simulink model "controllerTest"  (R2022b)
settings: Solver=ode45  StartTime=0  StopTime=T_f  MaxStep=MaxStep  RelTol=RelTol  AbsTol=1e-6
values from neighbouring files (symbols this model uses):
  A_ctrl = R_lti.A    [p62_inverted_pendulum.m]
  B_ctrl = R_lti.B    [p62_inverted_pendulum.m]
  beta = 0.1    [p62_inverted_pendulum.m]
  C_ctrl = R_lti.C    [p62_inverted_pendulum.m]
  D_ctrl = R_lti.D    [p62_inverted_pendulum.m]
  g = 9.81    [p62_inverted_pendulum.m]
  J_G = 0.006    [p62_inverted_pendulum.m]
  k = 0    [p62_inverted_pendulum.m]
  l = 0.6    [p62_inverted_pendulum.m]
  m = 0.2    [p62_inverted_pendulum.m]
  M = 0.5    [p62_inverted_pendulum.m]
  omega0 = 0    [p62_inverted_pendulum.m]
  theta0 = deg2rad(45)    [p62_inverted_pendulum.m]
  theta_ref = 0    [p62_inverted_pendulum.m]
  v0 = 0    [p62_inverted_pendulum.m]
  x0 = -5    [p62_inverted_pendulum.m]
Description:
  | Inverted Pendulum with Animation
  | 
  | This example shows how to model an inverted pendulum.  The animation is created using MATLAB(R) Handle Graphics(R).  The animation block is a masked
  | S-function.  For more information, use the context menu to look under the Animation block's mask
  | and open the S-function for editing.
settings Model: Creator=The MathWorks, Inc.  LastModifiedBy=alessandro
settings SolverCC: AutoScaleAbsTol=off  AlgebraicLoopSolver=TrustRegion
settings DataIOCC: ExternalInput=[]  InitialState=[]  SaveFormat=Array  SaveOutput=off  SaveTime=off  ReturnWorkspaceOutputs=off
settings OptimizationCC: BlockReduction=off  BooleanDataType=off  ExpressionDepthLimit=2147483647  InitFltsAndDblsToZero=on  LifeSpan=inf
settings DebuggingCC: SaveWithParameterizedLinksMsg=none  UnderspecifiedInitializationDetection=Classic  MergeDetectMultiDrivingBlocksExec=none  SignalResolutionControl=TryResolveAllWithWarning  MultiTaskDSMMsg=warning  MultiTaskCondExecSysMsg=none  SigSpecEnsureSampleTimeMsg=none  FcnCallInpInsideContextMsg=warning  UnconnectedInputMsg=warning  UnconnectedOutputMsg=warning  UnconnectedLineMsg=warning  StateNameClashWarn=warning  SFUnexpectedBacktrackingDiag=warning  SFNoUnconditionalDefaultTransitionDiag=warning  SFExecutionAtInitializationDiag=none  SFMachineParentedDataDiag=warning  ArithmeticOperatorsInVariantConditions=warning
settings HardwareCC: ProdBitPerPointer=32  ProdBitPerSizeT=32  ProdBitPerPtrDiffT=32  ProdLargestAtomicFloat=None  ProdIntDivRoundTo=Undefined  ProdEndianess=Unspecified  ProdWordSize=32  ProdHWDeviceType=32-bit Generic  TargetUnknown=on
settings ModelReferenceCC: EnableRefExpFcnMdlSchedulingChecks=on  PropagateSignalLabelsOutOfModel=off
settings SFSimCC: SimUseLocalCustomCode=off  CustomCodeUndefinedFunction=UseInterfaceOnly
settings RTWCC: RTWUseLocalCustomCode=off
settings CodeAppCC: StateflowObjectComments=on
settings GRTTargetCC: TargetFcnLib=ansi_tfl_tmw.mat  TargetLangStandard=C89/C90 (ANSI)  CombineOutputUpdateFcns=off  GRTInterface=on
settings ConfigComp: CovMetricSettings=dw  CovSaveCumulativeToWorkspaceVar=on  CovSaveSingleToWorkspaceVar=on  CovExternalEMLEnable=off

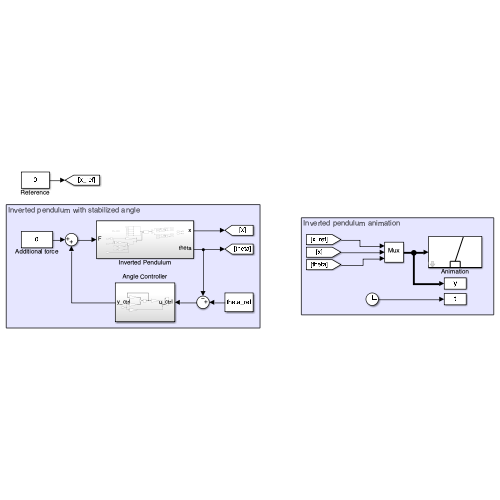
[thumbnail: Simulink's stored preview of the top-level diagram]
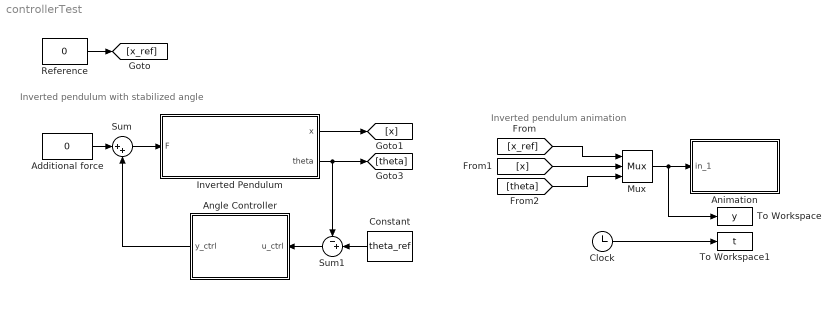
== system controllerTest ==
  note: Inverted pendulum with stabilized angle
  note: Inverted pendulum animation
  Additional force : Constant  Value=0
  Angle Controller : Subsystem
  Animation : Subsystem  mask(Pendulum plot){RefBlock=Reference}
      mask prompts: RefBlock "DC reference signal block name:"
      mask help: Pendulum plot
      mask Help: Pendulum animation function using Handle graphics.
      mask Display: plot([-10 10],[0 0],[-2 -2 2 2],[0 1 1 0],[0 3],[1 5])
  Clock : Clock
  Constant : Constant  Value=theta_ref
  Inverted Pendulum : Subsystem
  Mux : Mux  Inputs=3
  Reference : Constant  Value=0
  Sum : Sum  Inputs=|++
  Sum1 : Sum  Inputs=-+|
  To Workspace : ToWorkspace  VariableName=y  SampleTime=0.02
  To Workspace1 : ToWorkspace  VariableName=t  SampleTime=0.02
  wires:
  Reference/1 -> [x_ref]
  [x_ref] -> Mux/1
  [x] -> Mux/2
  [theta] -> Mux/3
  Mux/1 -> To Workspace/1, Animation/1(in_1)
  Clock/1 -> To Workspace1/1
  Inverted Pendulum/1(x) -> [x]
  Inverted Pendulum/2(theta) -> Sum1/1, [theta]
  Sum1/1 -> Angle Controller/1(u_ctrl)
  Angle Controller/1(y_ctrl) -> Sum/2
  Sum/1 -> Inverted Pendulum/1(F)
  Additional force/1 -> Sum/1
  Constant/1 -> Sum1/2

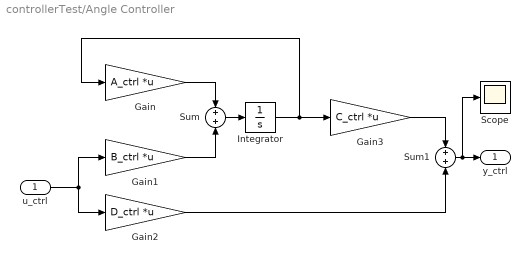
== system controllerTest/Angle Controller ==
  u_ctrl : Inport
  Gain : Gain  Gain=A_ctrl  Multiplication=Matrix(K*u)
  Gain1 : Gain  Gain=B_ctrl  Multiplication=Matrix(K*u)
  Gain2 : Gain  Gain=D_ctrl  Multiplication=Matrix(K*u)
  Gain3 : Gain  Gain=C_ctrl  Multiplication=Matrix(K*u)
  Integrator : Integrator
  Scope : Scope
  Sum : Sum
  Sum1 : Sum
  y_ctrl : Outport
  wires:
  Sum/1 -> Integrator/1
  Gain/1 -> Sum/1
  u_ctrl/1 -> Gain1/1, Gain2/1
  Integrator/1 -> Gain3/1, Gain/1
  Gain1/1 -> Sum/2
  Sum1/1 -> Scope/1, y_ctrl/1
  Gain3/1 -> Sum1/1
  Gain2/1 -> Sum1/2

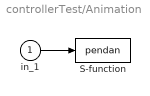
== system controllerTest/Animation ==
  in_1 : Inport
  S-function : S-Function  FunctionName=pendan  Parameters=RefBlock  SFunctionDeploymentMode=off  EnableBusSupport=off
      settings: DeleteFcn=pendan([],[],[],'DeleteBlock');
  wires:
  in_1/1 -> S-function/1

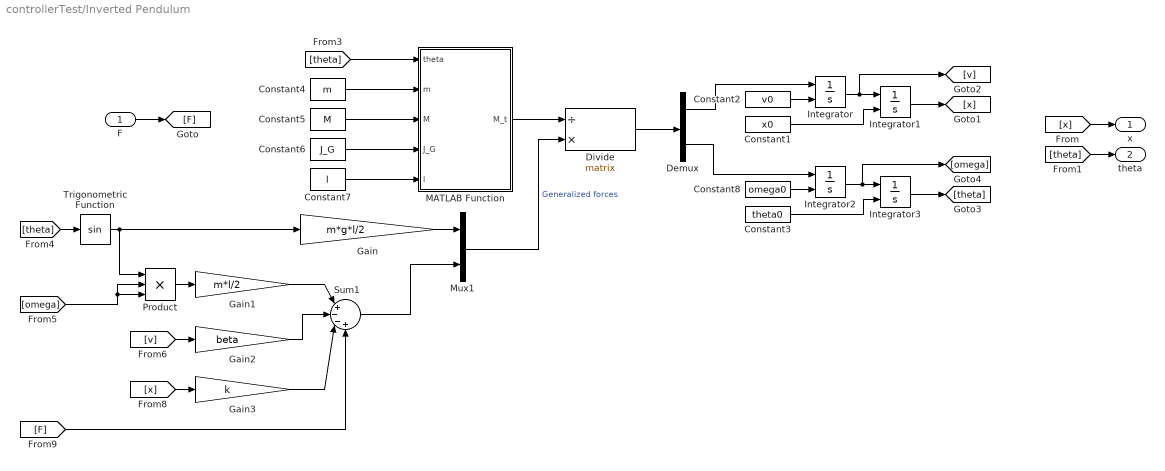
== system controllerTest/Inverted Pendulum ==
  F : Inport
  Constant1 : Constant  Value=x0
  Constant2 : Constant  Value=v0
  Constant3 : Constant  Value=theta0
  Constant4 : Constant  Value=m
  Constant5 : Constant  Value=M
  Constant6 : Constant  Value=J_G
  Constant7 : Constant  Value=l
  Constant8 : Constant  Value=omega0
  Demux : Demux  Outputs=2
  Divide : Product  Inputs=/*  Multiplication=Matrix(*)
  Gain : Gain  Gain=m*g*l/2
  Gain1 : Gain  Gain=m*l/2
  Gain2 : Gain  Gain=beta
  Gain3 : Gain  Gain=k
  Integrator : Integrator  InitialConditionSource=external
  Integrator1 : Integrator  InitialConditionSource=external
  Integrator2 : Integrator  InitialConditionSource=external
  Integrator3 : Integrator  InitialConditionSource=external  WrapState=on
  MATLAB Function : MATLAB Function  TreatAsAtomicUnit=on
  Mux1 : Mux  Inputs=2
  Product : Product  Inputs=3
  Sum1 : Sum  Inputs=|+--+
  Trigonometric Function : Trigonometry
  x : Outport
  theta : Outport  Port=2
  wires:
  Integrator/1 -> [v], Integrator1/1
  Integrator3/1 -> [theta]
  [theta] -> MATLAB Function/1(theta)
  [omega] -> Product/2, Product/3
  Integrator1/1 -> [x]
  Integrator2/1 -> [omega], Integrator3/1
  Divide/1 -> Demux/1
  Constant7/1 -> MATLAB Function/5(l)
  Demux/2 -> Integrator2/1
  Gain2/1 -> Sum1/2
  Constant5/1 -> MATLAB Function/3(M)
  Sum1/1 -> Mux1/2
  [theta] -> Trigonometric Function/1
  Constant6/1 -> MATLAB Function/4(J_G)
  Constant4/1 -> MATLAB Function/2(m)
  Product/1 -> Gain1/1
  MATLAB Function/1(M_t) -> Divide/1
  Gain/1 -> Mux1/1
  Trigonometric Function/1 -> Gain/1, Product/1
  Mux1/1 -> Divide/2  "Generalized forces"
  [F] -> Sum1/4
  Gain1/1 -> Sum1/1
  Constant2/1 -> Integrator/2
  Constant3/1 -> Integrator3/2
  [x] -> Gain3/1
  Demux/1 -> Integrator/1
  Gain3/1 -> Sum1/3
  [v] -> Gain2/1
  Constant1/1 -> Integrator1/2
  F/1 -> [F]
  [x] -> x/1
  [theta] -> theta/1
  Constant8/1 -> Integrator2/2

== matlab function controllerTest/Inverted Pendulum/MATLAB Function ==
  data: theta input; M_t output; m input; M input; J_G input; l input
function M_t = Inertia(theta, m, M, J_G, l)
%% Computation of the inertia matrix
M_t = [m*l/2*cos(theta)        J_G+m*l^2/4;
       M + m             m*l/2*cos(theta)];
